simulink model "test_matlabfcn_online"  (R2018a)
settings: Solver=FixedStepAuto  StartTime=0.0  StopTime=16000  FixedStep=100  RelTol=1e-3
InitFcn:
  | stop_time_as_str = get_param(gcs, 'StopTime');
  | stop_time = str2double(stop_time_as_str);
settings Model: Creator=gmb  LastModifiedBy=gmb

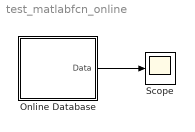
== system test_matlabfcn_online ==
  Online Database : Subsystem  mask{addr="127.0.0.1", port=3306, user="root", pass="", db="sim_test", tab="data", date_from="2018-04-17", time_from="06:00:00", date_until="2018-04-17", time_until="10:00:00", sensors="TW,I", interpolate=off}
      mask prompts: addr "Address"; user "Username"; pass "Password"; db "Database"; tab "Table"; date_from "Start day"; time_from "Start time"; date_until "End day"; time_until "End time"
  Scope : Scope
  wires:
  Online Database/1(Data) -> Scope/1

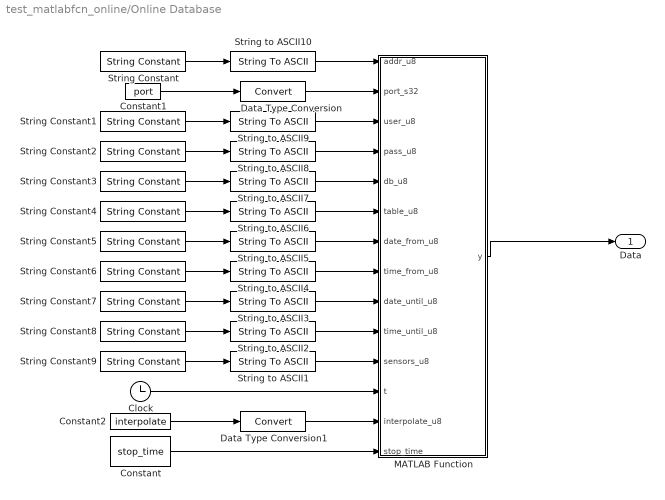
== system test_matlabfcn_online/Online Database ==
  Clock : Clock
  Constant : Constant  Value=stop_time
  Constant1 : Constant  Value=port
  Constant2 : Constant  Value=interpolate
  Data Type Conversion : DataTypeConversion
  Data Type Conversion1 : DataTypeConversion
  MATLAB Function : MATLAB Function  TreatAsAtomicUnit=on
  String Constant : StringConstant  String=addr
  String Constant1 : StringConstant  String=user
  String Constant2 : StringConstant  String=pass
  String Constant3 : StringConstant  String=db
  String Constant4 : StringConstant  String=tab
  String Constant5 : StringConstant  String=date_from
  String Constant6 : StringConstant  String=time_from
  String Constant7 : StringConstant  String=date_until
  String Constant8 : StringConstant  String=time_until
  String Constant9 : StringConstant  String=sensors
  String to ASCII{1..10} (10 alike) : StringToASCII
  Data : Outport
  wires:
  String Constant4/1 -> String to ASCII6/1
  String to ASCII1/1 -> MATLAB Function/11(sensors_u8)
  String Constant6/1 -> String to ASCII4/1
  String Constant/1 -> String to ASCII10/1
  Constant1/1 -> Data Type Conversion/1
  String Constant5/1 -> String to ASCII5/1
  String to ASCII5/1 -> MATLAB Function/7(date_from_u8)
  String to ASCII10/1 -> MATLAB Function/1(addr_u8)
  String Constant9/1 -> String to ASCII1/1
  String to ASCII7/1 -> MATLAB Function/5(db_u8)
  Clock/1 -> MATLAB Function/12(t)
  String to ASCII3/1 -> MATLAB Function/9(date_until_u8)
  String Constant7/1 -> String to ASCII3/1
  String to ASCII2/1 -> MATLAB Function/10(time_until_u8)
  String Constant2/1 -> String to ASCII8/1
  String to ASCII6/1 -> MATLAB Function/6(table_u8)
  String to ASCII9/1 -> MATLAB Function/3(user_u8)
  String to ASCII4/1 -> MATLAB Function/8(time_from_u8)
  String Constant3/1 -> String to ASCII7/1
  String to ASCII8/1 -> MATLAB Function/4(pass_u8)
  Constant/1 -> MATLAB Function/14(stop_time)
  Data Type Conversion/1 -> MATLAB Function/2(port_s32)
  String Constant1/1 -> String to ASCII9/1
  String Constant8/1 -> String to ASCII2/1
  MATLAB Function/1(y) -> Data/1
  Constant2/1 -> Data Type Conversion1/1
  Data Type Conversion1/1 -> MATLAB Function/13(interpolate_u8)

== matlab function test_matlabfcn_online/Online Database/MATLAB Function ==
  data: addr_u8 input; y output; port_s32 input; user_u8 input; pass_u8 input; db_u8 input; table_u8 input; date_from_u8 input; time_from_u8 input; date_until_u8 input; time_until_u8 input; sensors_u8 input; t input; interpolate_u8 input; stop_time input
function y = fcn(addr_u8, port_s32, user_u8, pass_u8, db_u8, table_u8, date_from_u8, time_from_u8, date_until_u8, time_until_u8, sensors_u8, t, interpolate_u8, stop_time)

persistent init;

coder.extrinsic('fullfile', 'loadlibrary', 'system_dependent', 'libfunctions','calllib','unloadlibrary', 'libpointer', 'resolve_pointer');

incpath = fullfile('c:\Program Files\','MySQL','MySQL Connector C 6.1','include');
[~, ~] = loadlibrary(['simdatabase',system_dependent('GetSharedLibExt')],'simdatabase.h', 'includepath', incpath);

if isempty(init)
   calllib('simdatabase','simdatabase_init');
   init = 1;
end

addr = char(addr_u8); 
user = char(user_u8);
pass = char(pass_u8);
db = char(db_u8);
table = char(table_u8);
date_from = char(date_from_u8);
time_from = char(time_from_u8);
date_until = char(date_until_u8);
time_until = char(time_until_u8);
sensors = char(sensors_u8);
interpolate = interpolate_u8;

vals = zeros(1, 10);
valPtr = libpointer('doublePtr', vals);
y = zeros(1, 10);

calllib('simdatabase','simdatabase_step_mysql', addr, port_s32, user, pass, db, table, date_from, time_from, date_until, time_until, sensors, t, interpolate, valPtr);

if(t >= stop_time)
   calllib('simdatabase','simdatabase_term');
   unloadlibrary('simdatabase');
end

y = resolve_pointer(valPtr);

end
